simulink model "ramadan_2022"  (R2021a)
settings: Solver=ode15s  StartTime=0.0  StopTime=10  MaxStep=1e-2  MinStep=1e-20  RelTol=1e-3
StartFcn:
  | tic
StopFcn:
  | toc
  | 
  | 
  | %if GimbalLockFlag
  |  % fprintf(2, 'Almost reached Gimbal Lock of IMU. Simulation stopped.\n')
  | %end
  | 
  | %fprintf('Elapsed time: %4.2f sec (%4.2f%% realtime)\n', a, tout(end)/a*100)
values from neighbouring files (symbols this model uses):
  Balance = pMod(26:29)    [AssignSimulinkParams.m]    (also in assign_parameters.m = param(26:29))
  BalanceTrunkLat = pMod(22:25)    [AssignSimulinkParams.m]    (also in assign_parameters.m = param(22:25))
  BasisStim = pMod(1:11)    [AssignSimulinkParams.m]    (also in assign_parameters.m = param(1:11))
  CompliantLeg = pMod(12:14)    [AssignSimulinkParams.m]    (also in assign_parameters.m = param(12:14))
  CompliantLegLat = pMod(15)    [AssignSimulinkParams.m]    (also in assign_parameters.m = param(15))
  lp1 = 0.45    [nms3D_prep.m]
  lp2 = 0.55    [nms3D_prep.m]
  N = size(x,1)    [cmaes_hg.m]
  PreventKneeOverextension = pMod(16:21)    [AssignSimulinkParams.m]    (also in assign_parameters.m = param(16:21))
  propulsion = pMod(35)    [AssignSimulinkParams.m]    (also in assign_parameters.m = param(35))
  s = x(1:N-1,:).^2 + x(2:N,:).^2    [cmaes_hg.m]
  Target02 = pMod(30)    [AssignSimulinkParams.m]    (also in assign_parameters.m = param(30))
  Target13 = pMod(31:33)    [AssignSimulinkParams.m]    (also in assign_parameters.m = param(31:33))
  theta0 = pMod(34)    [AssignSimulinkParams.m]    (also in assign_parameters.m = param(34))
  WramameiSL_1000 = readmatrix('WSL_1000_Norm_Sigmoid_MSE_cont.csv')    [nms3D_prep.m]
  ZramameiSL_1000 = readmatrix('ZSL_1000_Norm_Sigmoid_MSE_cont.csv')    [nms3D_prep.m]
undefined symbols (not defined in the file or in its folder): ICs, mParams, X, Y, Z
libraries: nesl_utility x110, sm_lib x88, simulink x79, eeGeneralControl x28, robotmaniplib x10, dspinverses x10, robotcorelib x5, dspmathops x3, pid_lib x2, vrlib x1
(part 8 of 9)

== system ramadan_2022/Supraspinal Level/Subsystem/Swing Leg/Compute Acceleration Profiles with Minimal Jerk Approach/Minimal jerk Hip Roll ==
  T_tot : Inport
  t_passed : Inport  Port=2
  "x0, dx0, ddx0" : Inport  Port=3
  "xT, dxT, ddxT" : Inport  Port=4
  Compare To Constant : simulink/Logic and Bit Operations/Compare To Constant  relop=>=  const=mParams.control.timelimit  OutDataTypeStr=boolean  ZeroCross=off
  Constant : Constant  Value=mParams.control.timelimit
  Constant1 : Constant  Value=0
  Demux : Demux  Outputs=3
  Demux1 : Demux  Outputs=3
  Enabled Subsystem : Subsystem  TreatAsAtomicUnit=on
  Minimal Jerk : Subsystem
  Minimal Jerk Parameters [Movellan] : Subsystem
  Minus : Sum  Inputs=+-
  Minus1 : Sum  Inputs=+-
  Switch : Switch
  jerk : Outport
  wires:
  Minimal Jerk/1(j(t)) -> jerk/1
  T_tot/1 -> Minus/1
  t_passed/1 -> Minus/2
  Constant1/1 -> Switch/1
  Demux/1 -> Minimal Jerk Parameters [Movellan]/1(x0)
  Demux/2 -> Minimal Jerk Parameters [Movellan]/2(dx0)
  Demux/3 -> Minimal Jerk Parameters [Movellan]/3(ddx0)
  Demux1/1 -> Minimal Jerk Parameters [Movellan]/4(xT)
  "x0, dx0, ddx0"/1 -> Demux/1
  Demux1/2 -> Minimal Jerk Parameters [Movellan]/5(dxT)
  "xT, dxT, ddxT"/1 -> Demux1/1
  Demux1/3 -> Minimal Jerk Parameters [Movellan]/6(ddxT)
  Minimal Jerk Parameters [Movellan]/1(a) -> Enabled Subsystem/1(In1)
  Minus/1 -> Compare To Constant/1, Minus1/2, Minimal Jerk Parameters [Movellan]/7(T)
  Enabled Subsystem/1(Out1) -> Minimal Jerk/2(a [6x1])
  Compare To Constant/1 -> Switch/2, Enabled Subsystem/Enable
  Constant/1 -> Minus1/1
  Minus1/1 -> Switch/3
  Switch/1 -> Minimal Jerk/1(t)

== system ramadan_2022/Supraspinal Level/Subsystem/Swing Leg/Compute Acceleration Profiles with Minimal Jerk Approach/Minimal jerk Hip Roll4 ==
  T_tot : Inport
  t_passed : Inport  Port=2
  "x0, dx0, ddx0" : Inport  Port=3
  "xT, dxT, ddxT" : Inport  Port=4
  Constant1 : Constant  Value=0
  Demux : Demux  Outputs=3
  Demux1 : Demux  Outputs=3
  Minimal Jerk : Subsystem
  Minimal Jerk Parameters[Movellan] : Subsystem
  Minus : Sum  Inputs=+-
  Saturation : Saturate  UpperLimit=inf  LowerLimit=0.08
  jerk : Outport
  wires:
  Minimal Jerk/1(j(t)) -> jerk/1
  T_tot/1 -> Minus/1
  Minimal Jerk Parameters[Movellan]/1(a) -> Minimal Jerk/2(a [6x1])
  t_passed/1 -> Minus/2
  Constant1/1 -> Minimal Jerk/1(t)
  Minus/1 -> Saturation/1
  Demux/1 -> Minimal Jerk Parameters[Movellan]/1(x0)
  Demux/2 -> Minimal Jerk Parameters[Movellan]/2(dx0)
  Demux/3 -> Minimal Jerk Parameters[Movellan]/3(ddx0)
  Demux1/1 -> Minimal Jerk Parameters[Movellan]/4(xT)
  "x0, dx0, ddx0"/1 -> Demux/1
  Demux1/2 -> Minimal Jerk Parameters[Movellan]/5(dxT)
  "xT, dxT, ddxT"/1 -> Demux1/1
  Demux1/3 -> Minimal Jerk Parameters[Movellan]/6(ddxT)
  Saturation/1 -> Minimal Jerk Parameters[Movellan]/7(T)

== system ramadan_2022/Supraspinal Level/Subsystem/Swing Leg/Compute Acceleration Profiles with Minimal Jerk Approach/Minimal jerk Knee ==
  T_tot : Inport
  t_passed : Inport  Port=2
  "x0, dx0, ddx0" : Inport  Port=3
  "xT, dxT, ddxT" : Inport  Port=4
  Compare To Constant1 : simulink/Logic and Bit Operations/Compare To Constant  relop=>=  const=mParams.control.timelimit  OutDataTypeStr=boolean  ZeroCross=off
  Constant : Constant  Value=mParams.control.timelimit
  Constant1 : Constant  Value=0
  Demux : Demux  Outputs=3
  Demux1 : Demux  Outputs=3
  Enabled Subsystem : Subsystem  TreatAsAtomicUnit=on
  Minimal Jerk : Subsystem
  Minimal Jerk Parameters [Movellan] : Subsystem
  Minus : Sum  Inputs=+-
  Minus1 : Sum  Inputs=+-
  Scope : Scope
  Scope1 : Scope  NumInputPorts=2
  Scope2 : Scope
  Switch : Switch
  jerk : Outport
  wires:
  Minimal Jerk/1(j(t)) -> jerk/1
  T_tot/1 -> Minus/1
  t_passed/1 -> Minus/2
  Constant1/1 -> Switch/1
  Demux/1 -> Scope1/1, Minimal Jerk Parameters [Movellan]/1(x0)
  Demux/2 -> Minimal Jerk Parameters [Movellan]/2(dx0)
  Demux/3 -> Minimal Jerk Parameters [Movellan]/3(ddx0)
  Demux1/1 -> Scope1/2, Minimal Jerk Parameters [Movellan]/4(xT)
  "x0, dx0, ddx0"/1 -> Demux/1
  Demux1/2 -> Minimal Jerk Parameters [Movellan]/5(dxT)
  "xT, dxT, ddxT"/1 -> Demux1/1
  Demux1/3 -> Minimal Jerk Parameters [Movellan]/6(ddxT)
  Minimal Jerk Parameters [Movellan]/1(a) -> Enabled Subsystem/1(In1)
  Minus/1 -> Scope/1, Compare To Constant1/1, Minus1/2, Minimal Jerk Parameters [Movellan]/7(T)
  Enabled Subsystem/1(Out1) -> Minimal Jerk/2(a [6x1])
  Compare To Constant1/1 -> Switch/2, Enabled Subsystem/Enable
  Constant/1 -> Minus1/1
  Minus1/1 -> Switch/3
  Switch/1 -> Minimal Jerk/1(t)

== system ramadan_2022/Supraspinal Level/Subsystem/Swing Leg/Compute Acceleration Profiles with Minimal Jerk Approach1/ Timer Phase 1 ==
  R : Inport
  Clock1 : Clock
  Clock3 : Clock
      settings: Decimation=4
  NOT : Logic  Operator=NOT  AllPortsSameDT=off  OutDataTypeStr=boolean
  Resettable Subsystem : Subsystem  TreatAsAtomicUnit=on
  Sum1 : Sum  Inputs=|+-  InputSameDT=on  SaturateOnIntegerOverflow=on  OutDataTypeStr=Inherit: Same as first input
  Switch2 : Switch  Criteria=u2 > Threshold  RndMeth=Zero
  t_passed : Outport  VectorParamsAs1DForOutWhenUnconnected=off
  wires:
  Clock1/1 -> Sum1/1
  Clock3/1 -> Switch2/3, Resettable Subsystem/1(In1)
  Sum1/1 -> t_passed/1
  R/1 -> NOT/1, Switch2/2
  Switch2/1 -> Sum1/2
  Resettable Subsystem/1(Out1) -> Switch2/1
  NOT/1 -> Resettable Subsystem/Enable

== system ramadan_2022/Supraspinal Level/Subsystem/Swing Leg/Compute Acceleration Profiles with Minimal Jerk Approach1/ Timer Phase 2 ==
  R : Inport
  Clock1 : Clock
  Clock3 : Clock
      settings: Decimation=4
  NOT : Logic  Operator=NOT  AllPortsSameDT=off  OutDataTypeStr=boolean
  Resettable Subsystem : Subsystem  TreatAsAtomicUnit=on
  Sum1 : Sum  Inputs=|+-  InputSameDT=on  SaturateOnIntegerOverflow=on  OutDataTypeStr=Inherit: Same as first input
  Switch2 : Switch  Criteria=u2 > Threshold  RndMeth=Zero
  Out : Outport  VectorParamsAs1DForOutWhenUnconnected=off
  wires:
  Clock1/1 -> Sum1/1
  Clock3/1 -> Switch2/3, Resettable Subsystem/1(In1)
  Sum1/1 -> Out/1
  R/1 -> NOT/1, Switch2/2
  Switch2/1 -> Sum1/2
  Resettable Subsystem/1(Out1) -> Switch2/1
  NOT/1 -> Resettable Subsystem/Enable

== system ramadan_2022/Supraspinal Level/Subsystem/Swing Leg/Compute Acceleration Profiles with Minimal Jerk Approach1/ Timer Phase 3 ==
  R : Inport
  Clock1 : Clock
  Clock3 : Clock
      settings: Decimation=4
  NOT : Logic  Operator=NOT  AllPortsSameDT=off  OutDataTypeStr=boolean
  Resettable Subsystem : Subsystem  TreatAsAtomicUnit=on
  Sum1 : Sum  Inputs=|+-  InputSameDT=on  SaturateOnIntegerOverflow=on  OutDataTypeStr=Inherit: Same as first input
  Switch2 : Switch  Criteria=u2 > Threshold  RndMeth=Zero
  t_passed : Outport  VectorParamsAs1DForOutWhenUnconnected=off
  wires:
  Clock1/1 -> Sum1/1
  Clock3/1 -> Switch2/3, Resettable Subsystem/1(In1)
  Sum1/1 -> t_passed/1
  R/1 -> NOT/1, Switch2/2
  Switch2/1 -> Sum1/2
  Resettable Subsystem/1(Out1) -> Switch2/1
  NOT/1 -> Resettable Subsystem/Enable

== system ramadan_2022/Supraspinal Level/Subsystem/Swing Leg/Compute Acceleration Profiles with Minimal Jerk Approach1/ Timer Phase 4 ==
  R : Inport
  Clock1 : Clock
  Clock3 : Clock
      settings: Decimation=4
  NOT : Logic  Operator=NOT  AllPortsSameDT=off  OutDataTypeStr=boolean
  Resettable Subsystem : Subsystem  TreatAsAtomicUnit=on
  Sum1 : Sum  Inputs=|+-  InputSameDT=on  SaturateOnIntegerOverflow=on  OutDataTypeStr=Inherit: Same as first input
  Switch2 : Switch  Criteria=u2 > Threshold  RndMeth=Zero
  t_passed : Outport  VectorParamsAs1DForOutWhenUnconnected=off
  wires:
  Clock1/1 -> Sum1/1
  Clock3/1 -> Switch2/3, Resettable Subsystem/1(In1)
  Sum1/1 -> t_passed/1
  R/1 -> NOT/1, Switch2/2
  Switch2/1 -> Sum1/2
  Resettable Subsystem/1(Out1) -> Switch2/1
  NOT/1 -> Resettable Subsystem/Enable

== system ramadan_2022/Supraspinal Level/Subsystem/Swing Leg/Compute Acceleration Profiles with Minimal Jerk Approach1/Minimal jerk Hip Roll4 ==
  T_tot : Inport
  t_passed : Inport  Port=2
  "x0, dx0, ddx0" : Inport  Port=3
  "xT, dxT, ddxT" : Inport  Port=4
  Constant1 : Constant  Value=0
  Demux : Demux  Outputs=3
  Demux1 : Demux  Outputs=3
  Minimal Jerk : Subsystem
  Minimal Jerk Parameters[Movellan] : Subsystem
  Minus : Sum  Inputs=+-
  Saturation : Saturate  UpperLimit=inf  LowerLimit=0.08
  jerk : Outport
  wires:
  Minimal Jerk/1(j(t)) -> jerk/1
  T_tot/1 -> Minus/1
  Minimal Jerk Parameters[Movellan]/1(a) -> Minimal Jerk/2(a [6x1])
  t_passed/1 -> Minus/2
  Constant1/1 -> Minimal Jerk/1(t)
  Minus/1 -> Saturation/1
  Demux/1 -> Minimal Jerk Parameters[Movellan]/1(x0)
  Demux/2 -> Minimal Jerk Parameters[Movellan]/2(dx0)
  Demux/3 -> Minimal Jerk Parameters[Movellan]/3(ddx0)
  Demux1/1 -> Minimal Jerk Parameters[Movellan]/4(xT)
  "x0, dx0, ddx0"/1 -> Demux/1
  Demux1/2 -> Minimal Jerk Parameters[Movellan]/5(dxT)
  "xT, dxT, ddxT"/1 -> Demux1/1
  Demux1/3 -> Minimal Jerk Parameters[Movellan]/6(ddxT)
  Saturation/1 -> Minimal Jerk Parameters[Movellan]/7(T)

== system ramadan_2022/Supraspinal Level/Subsystem/Swing Leg/Compute Acceleration Profiles with Minimal Jerk Approach1/Minimal jerk Leg Angle ==
  T_tot : Inport
  t_passed : Inport  Port=2
  "x0, dx0, ddx0" : Inport  Port=3
  "xT, dxT, ddxT" : Inport  Port=4
  Compare To Constant : simulink/Logic and Bit Operations/Compare To Constant  relop=>=  const=mParams.control.timelimit  OutDataTypeStr=boolean  ZeroCross=off
  Constant : Constant  Value=mParams.control.timelimit
  Constant1 : Constant  Value=0
  Demux : Demux  Outputs=3
  Demux1 : Demux  Outputs=3
  Enabled Subsystem : Subsystem  TreatAsAtomicUnit=on
  Minimal Jerk : Subsystem
  Minimal Jerk Parameters [Movellan] : Subsystem
  Minus : Sum  Inputs=+-
  Minus1 : Sum  Inputs=+-
  Switch : Switch
  jerk : Outport
  wires:
  Minimal Jerk/1(j(t)) -> jerk/1
  T_tot/1 -> Minus/1
  t_passed/1 -> Minus/2
  Constant1/1 -> Switch/1
  Demux/1 -> Minimal Jerk Parameters [Movellan]/1(x0)
  Demux/2 -> Minimal Jerk Parameters [Movellan]/2(dx0)
  Demux/3 -> Minimal Jerk Parameters [Movellan]/3(ddx0)
  Demux1/1 -> Minimal Jerk Parameters [Movellan]/4(xT)
  "x0, dx0, ddx0"/1 -> Demux/1
  Demux1/2 -> Minimal Jerk Parameters [Movellan]/5(dxT)
  "xT, dxT, ddxT"/1 -> Demux1/1
  Demux1/3 -> Minimal Jerk Parameters [Movellan]/6(ddxT)
  Minimal Jerk Parameters [Movellan]/1(a) -> Enabled Subsystem/1(In1)
  Minus/1 -> Compare To Constant/1, Minus1/2, Minimal Jerk Parameters [Movellan]/7(T)
  Enabled Subsystem/1(Out1) -> Minimal Jerk/2(a [6x1])
  Compare To Constant/1 -> Switch/2, Enabled Subsystem/Enable
  Constant/1 -> Minus1/1
  Minus1/1 -> Switch/3
  Switch/1 -> Minimal Jerk/1(t)

== system ramadan_2022/Supraspinal Level/Subsystem/Swing Leg/Compute Acceleration Profiles with Minimal Jerk Approach1/Minimal jerk Leg Length ==
  T_tot : Inport
  t_passed : Inport  Port=2
  "x0, dx0, ddx0" : Inport  Port=3
  "xT, dxT, ddxT" : Inport  Port=4
  Compare To Constant1 : simulink/Logic and Bit Operations/Compare To Constant  relop=>=  const=mParams.control.timelimit  OutDataTypeStr=boolean  ZeroCross=off
  Constant : Constant  Value=mParams.control.timelimit
  Constant1 : Constant  Value=0
  Demux : Demux  Outputs=3
  Demux1 : Demux  Outputs=3
  Enabled Subsystem : Subsystem  TreatAsAtomicUnit=on
  Minimal Jerk : Subsystem
  Minimal Jerk Parameters [Movellan] : Subsystem
  Minus : Sum  Inputs=+-
  Minus1 : Sum  Inputs=+-
  Switch : Switch
  jerk : Outport
  wires:
  Minimal Jerk/1(j(t)) -> jerk/1
  T_tot/1 -> Minus/1
  t_passed/1 -> Minus/2
  Constant1/1 -> Switch/1
  Demux/1 -> Minimal Jerk Parameters [Movellan]/1(x0)
  Demux/2 -> Minimal Jerk Parameters [Movellan]/2(dx0)
  Demux/3 -> Minimal Jerk Parameters [Movellan]/3(ddx0)
  Demux1/1 -> Minimal Jerk Parameters [Movellan]/4(xT)
  "x0, dx0, ddx0"/1 -> Demux/1
  Demux1/2 -> Minimal Jerk Parameters [Movellan]/5(dxT)
  "xT, dxT, ddxT"/1 -> Demux1/1
  Demux1/3 -> Minimal Jerk Parameters [Movellan]/6(ddxT)
  Minimal Jerk Parameters [Movellan]/1(a) -> Enabled Subsystem/1(In1)
  Minus/1 -> Compare To Constant1/1, Minus1/2, Minimal Jerk Parameters [Movellan]/7(T)
  Enabled Subsystem/1(Out1) -> Minimal Jerk/2(a [6x1])
  Compare To Constant1/1 -> Switch/2, Enabled Subsystem/Enable
  Constant/1 -> Minus1/1
  Minus1/1 -> Switch/3
  Switch/1 -> Minimal Jerk/1(t)

== system ramadan_2022/Supraspinal Level/Subsystem/Swing Leg/Compute Target States/Balance Control lateral ==
  Left/Right : Inport
  Constant : Constant  Value=0
  Constant1 : Constant
  Constant2 : Constant  Value=-1
  Divide : Product  Inputs=**
  Divide1 : Product  Inputs=**
  Minus5 : Sum  Inputs=+++
  Minus6 : Sum  Inputs=+-
  Product : Product
  Selector3 : Selector  InputPortWidth=3  IndexOptions=Index vector (dialog)  Indices=[3]  OutputSizes=1
  Selector4 : Selector  InputPortWidth=3  IndexOptions=Index vector (dialog)  Indices=[3]  OutputSizes=1
  Selector5 : Selector  InputPortWidth=3  IndexOptions=Index vector (dialog)  Indices=[3]  OutputSizes=1
  Switch : Switch  Criteria=u2 > Threshold
  Switch1 : Switch  Criteria=u2 > Threshold
  theta_Hip_swing_target : Outport
  wires:
  Divide/1 -> Minus5/2
  Switch/1 -> Minus6/2
  Divide1/1 -> Minus5/3
  [AnklePosR_rot] -> Selector3/1
  Minus6/1 -> Divide1/1
  Left/Right/1 -> Switch1/2, Switch/2
  [AnklePosL_rot] -> Selector4/1
  [cv_lat] -> Divide/2
  [cd_lat] -> Divide1/2
  Selector4/1 -> Switch/1
  Selector3/1 -> Switch/3
  [CoM_Velocity_rot] -> Selector5/1
  Selector5/1 -> Divide/1
  Constant/1 -> Minus6/1
  Minus5/1 -> theta_Hip_swing_target/1
  Product/1 -> Minus5/1
  [swh_lat] -> Product/2
  Switch1/1 -> Product/1
  Constant1/1 -> Switch1/1
  Constant2/1 -> Switch1/3

== system ramadan_2022/Supraspinal Level/Subsystem/Swing Leg/Compute Target States/Balance Control saggital ==
  Left/Right : Inport
  Constant : Constant  Value=0
  Divide : Product  Inputs=**
  Divide1 : Product  Inputs=**
  Minus5 : Sum  Inputs=+++
  Minus6 : Sum  Inputs=+-
  Selector3 : Selector  InputPortWidth=3  IndexOptions=Index vector (dialog)  Indices=[1]  OutputSizes=1
  Selector4 : Selector  InputPortWidth=3  IndexOptions=Index vector (dialog)  Indices=[1]  OutputSizes=1
  Selector5 : Selector  InputPortWidth=3  IndexOptions=Index vector (dialog)  Indices=[1]  OutputSizes=1
  Switch : Switch  Criteria=u2 > Threshold
  theta_Hip_swing_target : Outport
  tag scope: d=global
  wires:
  [swh] -> Minus5/1
  Switch/1 -> Minus6/2
  [AnklePosR_rot] -> Selector4/1
  Minus6/1 -> [d], Divide1/1
  Left/Right/1 -> Switch/2
  [AnklePosL_rot] -> Selector3/1
  [cv] -> Divide/2
  [cd] -> Divide1/2
  Divide/1 -> Minus5/2
  [CoM_Velocity_rot] -> Selector5/1
  Constant/1 -> Minus6/1
  Divide1/1 -> Minus5/3
  Minus5/1 -> theta_Hip_swing_target/1
  Selector5/1 -> Divide/1
  Selector3/1 -> Switch/1
  Selector4/1 -> Switch/3

== system ramadan_2022/Supraspinal Level/Subsystem/Swing Leg/Inverse Dynamics: Left Leg/Inverse Dynamics ==
  note: Augment Joint Vectors: In order to compute appropriate gravitational and velocity dependend forces, the joint angle and joint angle acceleration vectors are augmented by the position and velocity of the body in space.
  Joint Angles [rad] : Inport
  Joint Angle Velocities [rad/s] : Inport  Port=2
  Joint  Acceleration [rad/s^2] : Inport  Port=3
  Rotation Trunk [rad] : Inport  Port=4
  Trunk Position [m] : Inport  Port=5
  Rotation Velocity Trunk [rad/s] : Inport  Port=6
  Trunk Velocity [m/s] : Inport  Port=7
  Desired Acceleration [rad/s^2] : Inport  Port=8
  Enable : EnablePort  ZeroCross=off
  Constant : Constant  Value=zeros(6,1)
  Inverse Dynamics : Subsystem
  Mux : Mux  Inputs=3
  Mux1 : Mux  Inputs=3
  Mux2 : Mux  Inputs=2
  Mux4 : Mux  Inputs=2
  " Desired Torques" : Outport  VectorParamsAs1DForOutWhenUnconnected=off
  Interaction Wrench : Outport  Port=2  VectorParamsAs1DForOutWhenUnconnected=off
  wires:
  Trunk Position [m]/1 -> Mux1/1
  Inverse Dynamics/1(Desired Torques) -> " Desired Torques"/1
  Mux1/1 -> Inverse Dynamics/1(Config)
  Joint Angles [rad]/1 -> Mux1/3
  Rotation Trunk [rad]/1 -> Mux1/2
  Joint Angle Velocities [rad/s]/1 -> Mux/3
  Mux/1 -> Inverse Dynamics/2(JointVel)
  Desired Acceleration [rad/s^2]/1 -> Mux2/2
  Mux2/1 -> Inverse Dynamics/3(Des. JointAccel)
  Inverse Dynamics/2(Interaction Wrench Left) -> Interaction Wrench/1
  Constant/1 -> Mux4/1, Mux2/1
  Mux4/1 -> Inverse Dynamics/4(Real JointAccel)
  Joint  Acceleration [rad/s^2]/1 -> Mux4/2
  Trunk Velocity [m/s]/1 -> Mux/1
  Rotation Velocity Trunk [rad/s]/1 -> Mux/2

== system ramadan_2022/Supraspinal Level/Subsystem/Swing Leg/Inverse Dynamics: Left Leg/Sensor Data from Body Layer ==
  Constant : Constant  Commented=on  Value=0
  Constant1 : Constant  Value=zeros(3,1)
  From3 : From  Commented=on  GotoTag=TrunkRot_lat  TagVisibility=global
  From4 : From  Commented=on  GotoTag=TrunkRot_sag  TagVisibility=global
  From44 : From  Commented=on  GotoTag=RotationalVelocityTrunk  TagVisibility=global
  From46 : From  Commented=on  GotoTag=TranslationalVelocityTrunk  TagVisibility=global
  Gain : Gain  Gain=0
  Gain1 : Gain  Gain=0
  Mux : Mux  Commented=on  Inputs=3
  Scope : Scope
  Sensor Delay 1 : eeGeneralControl/Low-Pass Filter (Discrete or Continuous)  K=1  T=0.01  B=inf  A=-inf  init_option=Inherited from block input  x0=0  Ts=-1
  Sensor Delay 2 : eeGeneralControl/Low-Pass Filter (Discrete or Continuous)  K=1  T=0.01  B=inf  A=-inf  init_option=Inherited from block input  x0=0  Ts=-1
  Sensor Delay 3 : eeGeneralControl/Low-Pass Filter (Discrete or Continuous)  K=1  T=0.01  B=inf  A=-inf  init_option=Inherited from block input  x0=0  Ts=-1
  Joint Angles [rad] : Outport
  Joint Angle Velocities [rad/s] : Outport  Port=2
  Joint Angle Accelerations [rad/s^2] : Outport  Port=3
  " Rotation Trunk [rad]" : Outport  Port=4
  Trunk Position [m] : Outport  Port=5
  Rotation Velocity Trunk [rad/s] : Outport  Port=6
  Trunk Velocity [m/s] : Outport  Port=7
  wires:
  [Llegq] -> Sensor Delay 3/1
  [Llegdq] -> Sensor Delay 1/1
  Sensor Delay 3/1 -> Joint Angles [rad]/1
  Sensor Delay 1/1 -> Joint Angle Velocities [rad/s]/1
  [CoM_Position] -> Trunk Position [m]/1
  [Llegddq] -> Sensor Delay 2/1
  Sensor Delay 2/1 -> Joint Angle Accelerations [rad/s^2]/1, Scope/1
  From3/1 -> Mux/1
  Constant/1 -> Mux/2
  From4/1 -> Mux/3
  [RotationTrunk] -> " Rotation Trunk [rad]"/1
  Gain/1 -> Rotation Velocity Trunk [rad/s]/1
  Gain1/1 -> Trunk Velocity [m/s]/1
  Constant1/1 -> Gain1/1, Gain/1

== system ramadan_2022/Supraspinal Level/Subsystem/Swing Leg/Inverse Dynamics: Right Leg/Inverse Dynamics1 ==
  note: Augment Joint Vectors: In order to compute appropriate gravitational and velocity dependend forces, the joint angle and joint angle acceleration vectors are augmented by the position and velocity of the body in space.
  Joint Angles [rad] : Inport
  Joint Angle Velocities [rad/s] : Inport  Port=2
  Joint  Acceleration [rad/s^2] : Inport  Port=3
  Rotation Trunk [rad] : Inport  Port=4
  Trunk Position [m] : Inport  Port=5
  Rotation Velocity Trunk [rad/s] : Inport  Port=6
  Trunk Velocity [m/s] : Inport  Port=7
  Desired Acceleration [rad/s^2] : Inport  Port=8
  Enable : EnablePort  ZeroCross=off
  Constant : Constant  Value=zeros(6,1)
  Inverse Dynamics : Subsystem
  Mux : Mux  Inputs=3
  Mux1 : Mux  Inputs=3
  Mux2 : Mux  Inputs=2
  Mux4 : Mux  Inputs=2
  " Desired Torques" : Outport  VectorParamsAs1DForOutWhenUnconnected=off
  Interaction Wrench : Outport  Port=2  VectorParamsAs1DForOutWhenUnconnected=off
  wires:
  Trunk Position [m]/1 -> Mux1/1
  Inverse Dynamics/1(Desired Torques) -> " Desired Torques"/1
  Mux1/1 -> Inverse Dynamics/1(Config)
  Joint Angles [rad]/1 -> Mux1/3
  Rotation Trunk [rad]/1 -> Mux1/2
  Joint Angle Velocities [rad/s]/1 -> Mux/3
  Mux/1 -> Inverse Dynamics/2(JointVel)
  Desired Acceleration [rad/s^2]/1 -> Mux2/2
  Mux2/1 -> Inverse Dynamics/3(Des. JointAccel)
  Constant/1 -> Mux4/1, Mux2/1
  Mux4/1 -> Inverse Dynamics/4(Real JointAccel)
  Joint  Acceleration [rad/s^2]/1 -> Mux4/2
  Inverse Dynamics/2(Interaction Wrench Left) -> Interaction Wrench/1
  Trunk Velocity [m/s]/1 -> Mux/1
  Rotation Velocity Trunk [rad/s]/1 -> Mux/2

== system ramadan_2022/Supraspinal Level/Subsystem/Swing Leg/Inverse Dynamics: Right Leg/Sensor Data from Body Layer1 ==
  Constant1 : Constant  Value=zeros(3,1)
  From44 : From  Commented=on  GotoTag=RotationalVelocityTrunk  TagVisibility=global
  From46 : From  Commented=on  GotoTag=TranslationalVelocityTrunk  TagVisibility=global
  Gain : Gain  Gain=0
  Gain1 : Gain  Gain=0
  Sensor Delay 1 : eeGeneralControl/Low-Pass Filter (Discrete or Continuous)  K=1  T=0.01  B=inf  A=-inf  init_option=Inherited from block input  x0=0  Ts=-1
  Sensor Delay 2 : eeGeneralControl/Low-Pass Filter (Discrete or Continuous)  K=1  T=0.01  B=inf  A=-inf  init_option=Inherited from block input  x0=0  Ts=-1
  Sensor Delay 3 : eeGeneralControl/Low-Pass Filter (Discrete or Continuous)  K=1  T=0.01  B=inf  A=-inf  init_option=Inherited from block input  x0=0  Ts=-1
  Joint Angles [rad] : Outport
  Joint Angle Velocities [rad/s] : Outport  Port=2
  Joint Angle Accelerations [rad/s^2] : Outport  Port=3
  " Rotation Trunk [rad]" : Outport  Port=4
  Trunk Position [m] : Outport  Port=5
  Rotation Velocity Trunk [rad/s] : Outport  Port=6
  Trunk Velocity [m/s] : Outport  Port=7
  wires:
  [Rlegq] -> Sensor Delay 3/1
  [Rlegdq] -> Sensor Delay 1/1
  Sensor Delay 3/1 -> Joint Angles [rad]/1
  Sensor Delay 1/1 -> Joint Angle Velocities [rad/s]/1
  [CoM_Position] -> Trunk Position [m]/1
  [Rlegddq] -> Sensor Delay 2/1
  Sensor Delay 2/1 -> Joint Angle Accelerations [rad/s^2]/1
  [RotationTrunk] -> " Rotation Trunk [rad]"/1
  Gain/1 -> Rotation Velocity Trunk [rad/s]/1
  Gain1/1 -> Trunk Velocity [m/s]/1
  Constant1/1 -> Gain1/1, Gain/1

== system ramadan_2022/Supraspinal Level/Subsystem/Stance Leg2/Stance Leg/Inverse Dynamics Left Leg/Left Leg Ball ==
  Config : Inport
  Task : Inport  Port=2
  PD Input : Inport  Port=3
  Enable : EnablePort  ZeroCross=off
  Constant1 : Constant  Value="[0 0   ]"
  Gain : Gain
  Get Jacobian : robotmaniplib/Get Jacobian  RigidBodyTree=model_left_ball  EndEffector=EEF  SimulateUsing=Code generation
      settings: SourceProductBaseCode=RO
  Joint Space Mass Matrix : robotmaniplib/Joint Space Mass Matrix  RigidBodyTree=model_left_ball  SimulateUsing=Code generation
  Matrix Concatenate : Concatenate  Mode=Multidimensional array
  Matrix Multiply1 : Product  Multiplication=Matrix(*)
  Matrix Multiply4 : Product  Multiplication=Matrix(*)
  Mux2 : Mux  Inputs=3
  Pseudoinverse1 : dspinverses/Pseudoinverse  wanterr=off  SimulateUsing=Code generation
      settings: SourceProductBaseCode=DS
  Selector2 : Selector  NumberOfDimensions=2  InputPortWidth=3  IndexOptions=Index vector (dialog),Index vector (dialog)  Indices=mParams.control.constraints.pushoff,[1:5]  OutputSizes=1,1
  Selector3 : Selector  NumberOfDimensions=2  InputPortWidth=3  IndexOptions=Index vector (dialog),Index vector (dialog)  Indices="[1  4 ],[1:5]"  OutputSizes=1,1
  Push-Off Left (Ball) : Outport
  wires:
  Config/1 -> Get Jacobian/1, Joint Space Mass Matrix/1
  Selector2/1 -> Matrix Concatenate/1
  Pseudoinverse1/1 -> Matrix Multiply4/1
  Matrix Concatenate/1 -> Pseudoinverse1/1
  Selector3/1 -> Matrix Concatenate/2
  Constant1/1 -> Mux2/3
  Mux2/1 -> Matrix Multiply4/2
  Matrix Multiply1/1 -> Push-Off Left (Ball)/1
  Joint Space Mass Matrix/1 -> Matrix Multiply1/1, Selector3/1
  Get Jacobian/1 -> Selector2/1
  PD Input/1 -> Gain/1
  Matrix Multiply4/1 -> Matrix Multiply1/2
  Task/1 -> Mux2/1
  Gain/1 -> Mux2/2

== system ramadan_2022/Supraspinal Level/Subsystem/Stance Leg2/Stance Leg/Subsystem/Right Leg Ball ==
  Config : Inport
  Task : Inport  Port=2
  PD : Inport  Port=3
  Enable : EnablePort  ZeroCross=off
  Constant1 : Constant  Value="[0 0  ]"
  Get Jacobian : robotmaniplib/Get Jacobian  RigidBodyTree=model_right_ball  EndEffector=EEF  SimulateUsing=Code generation
      settings: SourceProductBaseCode=RO
  Joint Space Mass Matrix : robotmaniplib/Joint Space Mass Matrix  RigidBodyTree=model_right_ball  SimulateUsing=Code generation
  Matrix Concatenate : Concatenate  Mode=Multidimensional array
  Matrix Multiply1 : Product  Multiplication=Matrix(*)
  Matrix Multiply4 : Product  Multiplication=Matrix(*)
  Mux2 : Mux  Inputs=3
  Pseudoinverse1 : dspinverses/Pseudoinverse  wanterr=off  SimulateUsing=Code generation
      settings: SourceProductBaseCode=DS
  Selector2 : Selector  NumberOfDimensions=2  InputPortWidth=3  IndexOptions=Index vector (dialog),Index vector (dialog)  Indices=mParams.control.constraints.pushoff,[1:5]  OutputSizes=1,1
  Selector3 : Selector  NumberOfDimensions=2  InputPortWidth=3  IndexOptions=Index vector (dialog),Index vector (dialog)  Indices="[1  4 ],[1:5]"  OutputSizes=1,1
  Push-Off Right (Ball) : Outport
  wires:
  Matrix Multiply4/1 -> Matrix Multiply1/2
  Config/1 -> Get Jacobian/1, Joint Space Mass Matrix/1
  Selector2/1 -> Matrix Concatenate/1
  Pseudoinverse1/1 -> Matrix Multiply4/1
  Matrix Concatenate/1 -> Pseudoinverse1/1
  Selector3/1 -> Matrix Concatenate/2
  Constant1/1 -> Mux2/3
  Mux2/1 -> Matrix Multiply4/2
  Matrix Multiply1/1 -> Push-Off Right (Ball)/1
  Get Jacobian/1 -> Selector2/1
  Joint Space Mass Matrix/1 -> Matrix Multiply1/1, Selector3/1
  PD/1 -> Mux2/2
  Task/1 -> Mux2/1

== system ramadan_2022/Supraspinal Level/Subsystem/Swing Leg/Compute Acceleration Profiles with Minimal Jerk Approach/ Timer Phase 1/Resettable Subsystem ==
  In1 : Inport
  Enable : EnablePort  ZeroCross=off
  Out1 : Outport
  wires:
  In1/1 -> Out1/1

== system ramadan_2022/Supraspinal Level/Subsystem/Swing Leg/Compute Acceleration Profiles with Minimal Jerk Approach/ Timer Phase 2/Resettable Subsystem ==
  In1 : Inport
  Enable : EnablePort  ZeroCross=off
  Out1 : Outport
  wires:
  In1/1 -> Out1/1

== system ramadan_2022/Supraspinal Level/Subsystem/Swing Leg/Compute Acceleration Profiles with Minimal Jerk Approach/ Timer Phase 3/Resettable Subsystem ==
  In1 : Inport
  Enable : EnablePort  ZeroCross=off
  Out1 : Outport
  wires:
  In1/1 -> Out1/1

== system ramadan_2022/Supraspinal Level/Subsystem/Swing Leg/Compute Acceleration Profiles with Minimal Jerk Approach/ Timer Phase 4/Resettable Subsystem ==
  In1 : Inport
  Enable : EnablePort  ZeroCross=off
  Out1 : Outport
  wires:
  In1/1 -> Out1/1

== system ramadan_2022/Supraspinal Level/Subsystem/Swing Leg/Compute Acceleration Profiles with Minimal Jerk Approach/Minimal jerk Ankle/Enabled Subsystem ==
  In1 : Inport
  Enable : EnablePort
  Out1 : Outport  VectorParamsAs1DForOutWhenUnconnected=off
  wires:
  In1/1 -> Out1/1

== system ramadan_2022/Supraspinal Level/Subsystem/Swing Leg/Compute Acceleration Profiles with Minimal Jerk Approach/Minimal jerk Ankle/Minimal Jerk ==
  t : Inport
  a [6x1] : Inport  Port=2
  Add : Sum  Inputs=3
  Constant1 : Constant
  Constant3 : Constant  Value=2
  Demux : Demux  Outputs=6
  Divide3 : Product  Inputs=**
  Divide4 : Product  Inputs=**
  Divide5 : Product  Inputs=**
  Gain : Gain  Gain=60
  Gain1 : Gain  Gain=24
  Gain2 : Gain  Gain=6
  Math Function4 : Math  Operator=pow  SaturateOnIntegerOverflow=on
  Terminator : Terminator
  Terminator1 : Terminator
  Terminator2 : Terminator
  j(t) : Outport
  wires:
  a [6x1]/1 -> Demux/1
  Constant3/1 -> Math Function4/2
  Add/1 -> j(t)/1
  Demux/4 -> Divide3/2
  t/1 -> Divide4/1, Math Function4/1
  Demux/5 -> Divide4/2
  Demux/6 -> Divide5/2
  Demux/1 -> Terminator/1
  Demux/2 -> Terminator1/1
  Divide3/1 -> Gain2/1
  Divide4/1 -> Gain1/1
  Divide5/1 -> Gain/1
  Gain/1 -> Add/3
  Gain1/1 -> Add/2
  Gain2/1 -> Add/1
  Math Function4/1 -> Divide5/1
  Constant1/1 -> Divide3/1
  Demux/3 -> Terminator2/1

== system ramadan_2022/Supraspinal Level/Subsystem/Swing Leg/Compute Acceleration Profiles with Minimal Jerk Approach/Minimal jerk Ankle/Minimal Jerk Parameters [Movellan] ==
  x0 : Inport
  dx0 : Inport  Port=2
  ddx0 : Inport  Port=3
  xT : Inport  Port=4
  dxT : Inport  Port=5
  ddxT : Inport  Port=6
  T : Inport  Port=7
  Demux : Demux  Outputs=3
  Gain : Gain  Gain=0.5
  Gain1 : Gain  Gain=3
  Gain2 : Gain  Gain=6
  Gain3 : Gain  Gain=4
  Gain4 : Gain  Gain=12
  Gain5 : Gain  Gain=5
  Gain6 : Gain  Gain=20
  Matrix Multiply : Product  Multiplication=Matrix(*)
  Minus : Sum  Inputs=+---
  Minus1 : Sum  Inputs=+--
  Minus2 : Sum  Inputs=+-
  Mux : Mux  Inputs=6
  Mux{1..4} (4 alike) : Mux  Inputs=3
  Pseudoinverse : dspinverses/Pseudoinverse  wanterr=off  SimulateUsing=Code generation
      settings: SourceProductBaseCode=DS
  T{2..5} (4 alike) : Product  Inputs=**
  b : Concatenate  NumInputs=3  Mode=Multidimensional array  ConcatenateDimension=2
  multiply : Product  Inputs=**
  multiply1 : Product  Inputs=**
  multiply2 : Product  Inputs=**
  a : Outport
  wires:
  xT/1 -> Minus/1
  Minus1/1 -> Mux4/2
  T5/1 -> Mux3/1
  multiply1/1 -> Minus1/3
  Gain5/1 -> Mux3/2
  Demux/2 -> Mux/5
  dxT/1 -> Minus1/1
  Demux/3 -> Mux/6
  b/1 -> Pseudoinverse/1
  multiply2/1 -> Minus/3
  Minus2/1 -> Mux4/3
  Gain/1 -> multiply/1, Mux/3
  multiply/1 -> Minus/4
  ddxT/1 -> Minus2/1
  Gain4/1 -> Mux2/3
  Gain6/1 -> Mux3/3
  x0/1 -> Minus/2, Mux/1
  Mux1/1 -> b/1
  Matrix Multiply/1 -> Demux/1
  ddx0/1 -> Minus2/2, multiply1/1, Gain/1
  T2/1 -> Gain1/1, Gain4/1, T3/1, multiply/2
  Gain2/1 -> Mux1/3
  Mux4/1 -> Matrix Multiply/2
  T4/1 -> Mux2/1, Gain5/1, T5/1
  Minus/1 -> Mux4/1
  Pseudoinverse/1 -> Matrix Multiply/1
  Mux2/1 -> b/2
  Gain3/1 -> Mux2/2
  Mux3/1 -> b/3
  Gain1/1 -> Mux1/2
  T/1 -> multiply2/2, multiply1/2, Gain2/1, T5/2, T4/2, T3/2, T2/2, T2/1
  Demux/1 -> Mux/4
  Mux/1 -> a/1
  T3/1 -> Gain6/1, Gain3/1, Mux1/1, T4/1
  dx0/1 -> multiply2/1, Minus1/2, Mux/2

== system ramadan_2022/Supraspinal Level/Subsystem/Swing Leg/Compute Acceleration Profiles with Minimal Jerk Approach/Minimal jerk Hip Pitch/Enabled Subsystem ==
  In1 : Inport
  Enable : EnablePort
  Out1 : Outport  VectorParamsAs1DForOutWhenUnconnected=off
  wires:
  In1/1 -> Out1/1

== system ramadan_2022/Supraspinal Level/Subsystem/Swing Leg/Compute Acceleration Profiles with Minimal Jerk Approach/Minimal jerk Hip Pitch/Minimal Jerk ==
  t : Inport
  a [6x1] : Inport  Port=2
  Add : Sum  Inputs=3
  Constant1 : Constant
  Constant3 : Constant  Value=2
  Demux : Demux  Outputs=6
  Divide3 : Product  Inputs=**
  Divide4 : Product  Inputs=**
  Divide5 : Product  Inputs=**
  Gain : Gain  Gain=60
  Gain1 : Gain  Gain=24
  Gain2 : Gain  Gain=6
  Math Function4 : Math  Operator=pow  SaturateOnIntegerOverflow=on
  Terminator : Terminator
  Terminator1 : Terminator
  Terminator2 : Terminator
  j(t) : Outport
  wires:
  a [6x1]/1 -> Demux/1
  Constant3/1 -> Math Function4/2
  Add/1 -> j(t)/1
  Demux/4 -> Divide3/2
  t/1 -> Divide4/1, Math Function4/1
  Demux/5 -> Divide4/2
  Demux/6 -> Divide5/2
  Demux/1 -> Terminator/1
  Demux/2 -> Terminator1/1
  Divide3/1 -> Gain2/1
  Divide4/1 -> Gain1/1
  Divide5/1 -> Gain/1
  Gain/1 -> Add/3
  Gain1/1 -> Add/2
  Gain2/1 -> Add/1
  Math Function4/1 -> Divide5/1
  Constant1/1 -> Divide3/1
  Demux/3 -> Terminator2/1

== system ramadan_2022/Supraspinal Level/Subsystem/Swing Leg/Compute Acceleration Profiles with Minimal Jerk Approach/Minimal jerk Hip Pitch/Minimal Jerk Parameters [Movellan] ==
  x0 : Inport
  dx0 : Inport  Port=2
  ddx0 : Inport  Port=3
  xT : Inport  Port=4
  dxT : Inport  Port=5
  ddxT : Inport  Port=6
  T : Inport  Port=7
  Demux : Demux  Outputs=3
  Gain : Gain  Gain=0.5
  Gain1 : Gain  Gain=3
  Gain2 : Gain  Gain=6
  Gain3 : Gain  Gain=4
  Gain4 : Gain  Gain=12
  Gain5 : Gain  Gain=5
  Gain6 : Gain  Gain=20
  Matrix Multiply : Product  Multiplication=Matrix(*)
  Minus : Sum  Inputs=+---
  Minus1 : Sum  Inputs=+--
  Minus2 : Sum  Inputs=+-
  Mux : Mux  Inputs=6
  Mux{1..4} (4 alike) : Mux  Inputs=3
  Pseudoinverse : dspinverses/Pseudoinverse  wanterr=off  SimulateUsing=Code generation
      settings: SourceProductBaseCode=DS
  T{2..5} (4 alike) : Product  Inputs=**
  b : Concatenate  NumInputs=3  Mode=Multidimensional array  ConcatenateDimension=2
  multiply : Product  Inputs=**
  multiply1 : Product  Inputs=**
  multiply2 : Product  Inputs=**
  a : Outport
  wires:
  xT/1 -> Minus/1
  Minus1/1 -> Mux4/2
  T5/1 -> Mux3/1
  multiply1/1 -> Minus1/3
  Gain5/1 -> Mux3/2
  Demux/2 -> Mux/5
  dxT/1 -> Minus1/1
  Demux/3 -> Mux/6
  b/1 -> Pseudoinverse/1
  multiply2/1 -> Minus/3
  Minus2/1 -> Mux4/3
  Gain/1 -> multiply/1, Mux/3
  multiply/1 -> Minus/4
  ddxT/1 -> Minus2/1
  Gain4/1 -> Mux2/3
  Gain6/1 -> Mux3/3
  x0/1 -> Minus/2, Mux/1
  Mux1/1 -> b/1
  Matrix Multiply/1 -> Demux/1
  ddx0/1 -> Minus2/2, multiply1/1, Gain/1
  T2/1 -> Gain1/1, Gain4/1, T3/1, multiply/2
  Gain2/1 -> Mux1/3
  Mux4/1 -> Matrix Multiply/2
  T4/1 -> Mux2/1, Gain5/1, T5/1
  Minus/1 -> Mux4/1
  Pseudoinverse/1 -> Matrix Multiply/1
  Mux2/1 -> b/2
  Gain3/1 -> Mux2/2
  Mux3/1 -> b/3
  Gain1/1 -> Mux1/2
  T/1 -> multiply2/2, multiply1/2, Gain2/1, T5/2, T4/2, T3/2, T2/2, T2/1
  Demux/1 -> Mux/4
  Mux/1 -> a/1
  T3/1 -> Gain6/1, Gain3/1, Mux1/1, T4/1
  dx0/1 -> multiply2/1, Minus1/2, Mux/2

== system ramadan_2022/Supraspinal Level/Subsystem/Swing Leg/Compute Acceleration Profiles with Minimal Jerk Approach/Minimal jerk Hip Roll/Enabled Subsystem ==
  In1 : Inport
  Enable : EnablePort
  Out1 : Outport  VectorParamsAs1DForOutWhenUnconnected=off
  wires:
  In1/1 -> Out1/1

== system ramadan_2022/Supraspinal Level/Subsystem/Swing Leg/Compute Acceleration Profiles with Minimal Jerk Approach/Minimal jerk Hip Roll/Minimal Jerk ==
  t : Inport
  a [6x1] : Inport  Port=2
  Add : Sum  Inputs=3
  Constant1 : Constant
  Constant3 : Constant  Value=2
  Demux : Demux  Outputs=6
  Divide3 : Product  Inputs=**
  Divide4 : Product  Inputs=**
  Divide5 : Product  Inputs=**
  Gain : Gain  Gain=60
  Gain1 : Gain  Gain=24
  Gain2 : Gain  Gain=6
  Math Function4 : Math  Operator=pow  SaturateOnIntegerOverflow=on
  Terminator : Terminator
  Terminator1 : Terminator
  Terminator2 : Terminator
  j(t) : Outport
  wires:
  a [6x1]/1 -> Demux/1
  Constant3/1 -> Math Function4/2
  Add/1 -> j(t)/1
  Demux/4 -> Divide3/2
  t/1 -> Divide4/1, Math Function4/1
  Demux/5 -> Divide4/2
  Demux/6 -> Divide5/2
  Demux/1 -> Terminator/1
  Demux/2 -> Terminator1/1
  Divide3/1 -> Gain2/1
  Divide4/1 -> Gain1/1
  Divide5/1 -> Gain/1
  Gain/1 -> Add/3
  Gain1/1 -> Add/2
  Gain2/1 -> Add/1
  Math Function4/1 -> Divide5/1
  Constant1/1 -> Divide3/1
  Demux/3 -> Terminator2/1

== system ramadan_2022/Supraspinal Level/Subsystem/Swing Leg/Compute Acceleration Profiles with Minimal Jerk Approach/Minimal jerk Hip Roll/Minimal Jerk Parameters [Movellan] ==
  x0 : Inport
  dx0 : Inport  Port=2
  ddx0 : Inport  Port=3
  xT : Inport  Port=4
  dxT : Inport  Port=5
  ddxT : Inport  Port=6
  T : Inport  Port=7
  Demux : Demux  Outputs=3
  Gain : Gain  Gain=0.5
  Gain1 : Gain  Gain=3
  Gain2 : Gain  Gain=6
  Gain3 : Gain  Gain=4
  Gain4 : Gain  Gain=12
  Gain5 : Gain  Gain=5
  Gain6 : Gain  Gain=20
  Matrix Multiply : Product  Multiplication=Matrix(*)
  Minus : Sum  Inputs=+---
  Minus1 : Sum  Inputs=+--
  Minus2 : Sum  Inputs=+-
  Mux : Mux  Inputs=6
  Mux{1..4} (4 alike) : Mux  Inputs=3
  Pseudoinverse : dspinverses/Pseudoinverse  wanterr=off  SimulateUsing=Code generation
      settings: SourceProductBaseCode=DS
  T{2..5} (4 alike) : Product  Inputs=**
  b : Concatenate  NumInputs=3  Mode=Multidimensional array  ConcatenateDimension=2
  multiply : Product  Inputs=**
  multiply1 : Product  Inputs=**
  multiply2 : Product  Inputs=**
  a : Outport
  wires:
  xT/1 -> Minus/1
  Minus1/1 -> Mux4/2
  T5/1 -> Mux3/1
  multiply1/1 -> Minus1/3
  Gain5/1 -> Mux3/2
  Demux/2 -> Mux/5
  dxT/1 -> Minus1/1
  Demux/3 -> Mux/6
  b/1 -> Pseudoinverse/1
  multiply2/1 -> Minus/3
  Minus2/1 -> Mux4/3
  Gain/1 -> multiply/1, Mux/3
  multiply/1 -> Minus/4
  ddxT/1 -> Minus2/1
  Gain4/1 -> Mux2/3
  Gain6/1 -> Mux3/3
  x0/1 -> Minus/2, Mux/1
  Mux1/1 -> b/1
  Matrix Multiply/1 -> Demux/1
  ddx0/1 -> Minus2/2, multiply1/1, Gain/1
  T2/1 -> Gain1/1, Gain4/1, T3/1, multiply/2
  Gain2/1 -> Mux1/3
  Mux4/1 -> Matrix Multiply/2
  T4/1 -> Mux2/1, Gain5/1, T5/1
  Minus/1 -> Mux4/1
  Pseudoinverse/1 -> Matrix Multiply/1
  Mux2/1 -> b/2
  Gain3/1 -> Mux2/2
  Mux3/1 -> b/3
  Gain1/1 -> Mux1/2
  T/1 -> multiply2/2, multiply1/2, Gain2/1, T5/2, T4/2, T3/2, T2/2, T2/1
  Demux/1 -> Mux/4
  Mux/1 -> a/1
  T3/1 -> Gain6/1, Gain3/1, Mux1/1, T4/1
  dx0/1 -> multiply2/1, Minus1/2, Mux/2

== system ramadan_2022/Supraspinal Level/Subsystem/Swing Leg/Compute Acceleration Profiles with Minimal Jerk Approach/Minimal jerk Hip Roll4/Minimal Jerk ==
  t : Inport
  a [6x1] : Inport  Port=2
  Add : Sum  Inputs=3
  Constant1 : Constant
  Constant3 : Constant  Value=2
  Demux : Demux  Outputs=6
  Divide3 : Product  Inputs=**
  Divide4 : Product  Inputs=**
  Divide5 : Product  Inputs=**
  Gain : Gain  Gain=60
  Gain1 : Gain  Gain=24
  Gain2 : Gain  Gain=6
  Math Function4 : Math  Operator=pow  SaturateOnIntegerOverflow=on
  Terminator : Terminator
  Terminator1 : Terminator
  Terminator2 : Terminator
  j(t) : Outport
  wires:
  a [6x1]/1 -> Demux/1
  Constant3/1 -> Math Function4/2
  Add/1 -> j(t)/1
  Demux/4 -> Divide3/2
  t/1 -> Divide4/1, Math Function4/1
  Demux/5 -> Divide4/2
  Demux/6 -> Divide5/2
  Demux/1 -> Terminator/1
  Demux/2 -> Terminator1/1
  Divide3/1 -> Gain2/1
  Divide4/1 -> Gain1/1
  Divide5/1 -> Gain/1
  Gain/1 -> Add/3
  Gain1/1 -> Add/2
  Gain2/1 -> Add/1
  Math Function4/1 -> Divide5/1
  Constant1/1 -> Divide3/1
  Demux/3 -> Terminator2/1

== system ramadan_2022/Supraspinal Level/Subsystem/Swing Leg/Compute Acceleration Profiles with Minimal Jerk Approach/Minimal jerk Hip Roll4/Minimal Jerk Parameters[Movellan] ==
  x0 : Inport
  dx0 : Inport  Port=2
  ddx0 : Inport  Port=3
  xT : Inport  Port=4
  dxT : Inport  Port=5
  ddxT : Inport  Port=6
  T : Inport  Port=7
  Demux : Demux  Outputs=3
  Gain : Gain  Gain=0.5
  Gain1 : Gain  Gain=3
  Gain2 : Gain  Gain=6
  Gain3 : Gain  Gain=4
  Gain4 : Gain  Gain=12
  Gain5 : Gain  Gain=5
  Gain6 : Gain  Gain=20
  Matrix Multiply : Product  Multiplication=Matrix(*)
  Minus : Sum  Inputs=+---
  Minus1 : Sum  Inputs=+--
  Minus2 : Sum  Inputs=+-
  Mux : Mux  Inputs=6
  Mux{1..4} (4 alike) : Mux  Inputs=3
  Pseudoinverse : dspinverses/Pseudoinverse  wanterr=off  SimulateUsing=Code generation
      settings: SourceProductBaseCode=DS
  T{2..5} (4 alike) : Product  Inputs=**
  b : Concatenate  NumInputs=3  Mode=Multidimensional array  ConcatenateDimension=2
  multiply : Product  Inputs=**
  multiply1 : Product  Inputs=**
  multiply2 : Product  Inputs=**
  a : Outport
  wires:
  xT/1 -> Minus/1
  Minus1/1 -> Mux4/2
  T5/1 -> Mux3/1
  multiply1/1 -> Minus1/3
  Gain5/1 -> Mux3/2
  Demux/2 -> Mux/5
  dxT/1 -> Minus1/1
  Demux/3 -> Mux/6
  b/1 -> Pseudoinverse/1
  multiply2/1 -> Minus/3
  Minus2/1 -> Mux4/3
  Gain/1 -> multiply/1, Mux/3
  multiply/1 -> Minus/4
  ddxT/1 -> Minus2/1
  Gain4/1 -> Mux2/3
  Gain6/1 -> Mux3/3
  x0/1 -> Minus/2, Mux/1
  Mux1/1 -> b/1
  Matrix Multiply/1 -> Demux/1
  ddx0/1 -> Minus2/2, multiply1/1, Gain/1
  T2/1 -> Gain1/1, Gain4/1, T3/1, multiply/2
  Gain2/1 -> Mux1/3
  Mux4/1 -> Matrix Multiply/2
  T4/1 -> Mux2/1, Gain5/1, T5/1
  Minus/1 -> Mux4/1
  Pseudoinverse/1 -> Matrix Multiply/1
  Mux2/1 -> b/2
  Gain3/1 -> Mux2/2
  Mux3/1 -> b/3
  Gain1/1 -> Mux1/2
  T/1 -> multiply2/2, multiply1/2, Gain2/1, T5/2, T4/2, T3/2, T2/2, T2/1
  Demux/1 -> Mux/4
  Mux/1 -> a/1
  T3/1 -> Gain6/1, Gain3/1, Mux1/1, T4/1
  dx0/1 -> multiply2/1, Minus1/2, Mux/2

== system ramadan_2022/Supraspinal Level/Subsystem/Swing Leg/Compute Acceleration Profiles with Minimal Jerk Approach/Minimal jerk Knee/Enabled Subsystem ==
  In1 : Inport
  Enable : EnablePort
  Out1 : Outport  VectorParamsAs1DForOutWhenUnconnected=off
  wires:
  In1/1 -> Out1/1

== system ramadan_2022/Supraspinal Level/Subsystem/Swing Leg/Compute Acceleration Profiles with Minimal Jerk Approach/Minimal jerk Knee/Minimal Jerk ==
  t : Inport
  a [6x1] : Inport  Port=2
  Add : Sum  Inputs=3
  Constant1 : Constant
  Constant3 : Constant  Value=2
  Demux : Demux  Outputs=6
  Divide3 : Product  Inputs=**
  Divide4 : Product  Inputs=**
  Divide5 : Product  Inputs=**
  Gain : Gain  Gain=60
  Gain1 : Gain  Gain=24
  Gain2 : Gain  Gain=6
  Math Function4 : Math  Operator=pow  SaturateOnIntegerOverflow=on
  Terminator : Terminator
  Terminator1 : Terminator
  Terminator2 : Terminator
  j(t) : Outport
  wires:
  a [6x1]/1 -> Demux/1
  Constant3/1 -> Math Function4/2
  Add/1 -> j(t)/1
  Demux/4 -> Divide3/2
  t/1 -> Divide4/1, Math Function4/1
  Demux/5 -> Divide4/2
  Demux/6 -> Divide5/2
  Demux/1 -> Terminator/1
  Demux/2 -> Terminator1/1
  Divide3/1 -> Gain2/1
  Divide4/1 -> Gain1/1
  Divide5/1 -> Gain/1
  Gain/1 -> Add/3
  Gain1/1 -> Add/2
  Gain2/1 -> Add/1
  Math Function4/1 -> Divide5/1
  Constant1/1 -> Divide3/1
  Demux/3 -> Terminator2/1

== system ramadan_2022/Supraspinal Level/Subsystem/Swing Leg/Compute Acceleration Profiles with Minimal Jerk Approach/Minimal jerk Knee/Minimal Jerk Parameters [Movellan] ==
  x0 : Inport
  dx0 : Inport  Port=2
  ddx0 : Inport  Port=3
  xT : Inport  Port=4
  dxT : Inport  Port=5
  ddxT : Inport  Port=6
  T : Inport  Port=7
  Demux : Demux  Outputs=3
  Gain : Gain  Gain=0.5
  Gain1 : Gain  Gain=3
  Gain2 : Gain  Gain=6
  Gain3 : Gain  Gain=4
  Gain4 : Gain  Gain=12
  Gain5 : Gain  Gain=5
  Gain6 : Gain  Gain=20
  Matrix Multiply : Product  Multiplication=Matrix(*)
  Minus : Sum  Inputs=+---
  Minus1 : Sum  Inputs=+--
  Minus2 : Sum  Inputs=+-
  Mux : Mux  Inputs=6
  Mux{1..4} (4 alike) : Mux  Inputs=3
  Pseudoinverse : dspinverses/Pseudoinverse  wanterr=off  SimulateUsing=Code generation
      settings: SourceProductBaseCode=DS
  T{2..5} (4 alike) : Product  Inputs=**
  b : Concatenate  NumInputs=3  Mode=Multidimensional array  ConcatenateDimension=2
  multiply : Product  Inputs=**
  multiply1 : Product  Inputs=**
  multiply2 : Product  Inputs=**
  a : Outport
  wires:
  xT/1 -> Minus/1
  Minus1/1 -> Mux4/2
  T5/1 -> Mux3/1
  multiply1/1 -> Minus1/3
  Gain5/1 -> Mux3/2
  Demux/2 -> Mux/5
  dxT/1 -> Minus1/1
  Demux/3 -> Mux/6
  b/1 -> Pseudoinverse/1
  multiply2/1 -> Minus/3
  Minus2/1 -> Mux4/3
  Gain/1 -> multiply/1, Mux/3
  multiply/1 -> Minus/4
  ddxT/1 -> Minus2/1
  Gain4/1 -> Mux2/3
  Gain6/1 -> Mux3/3
  x0/1 -> Minus/2, Mux/1
  Mux1/1 -> b/1
  Matrix Multiply/1 -> Demux/1
  ddx0/1 -> Minus2/2, multiply1/1, Gain/1
  T2/1 -> Gain1/1, Gain4/1, T3/1, multiply/2
  Gain2/1 -> Mux1/3
  Mux4/1 -> Matrix Multiply/2
  T4/1 -> Mux2/1, Gain5/1, T5/1
  Minus/1 -> Mux4/1
  Pseudoinverse/1 -> Matrix Multiply/1
  Mux2/1 -> b/2
  Gain3/1 -> Mux2/2
  Mux3/1 -> b/3
  Gain1/1 -> Mux1/2
  T/1 -> multiply2/2, multiply1/2, Gain2/1, T5/2, T4/2, T3/2, T2/2, T2/1
  Demux/1 -> Mux/4
  Mux/1 -> a/1
  T3/1 -> Gain6/1, Gain3/1, Mux1/1, T4/1
  dx0/1 -> multiply2/1, Minus1/2, Mux/2

== system ramadan_2022/Supraspinal Level/Subsystem/Swing Leg/Compute Acceleration Profiles with Minimal Jerk Approach1/ Timer Phase 1/Resettable Subsystem ==
  In1 : Inport
  Enable : EnablePort  ZeroCross=off
  Out1 : Outport
  wires:
  In1/1 -> Out1/1

== system ramadan_2022/Supraspinal Level/Subsystem/Swing Leg/Compute Acceleration Profiles with Minimal Jerk Approach1/ Timer Phase 2/Resettable Subsystem ==
  In1 : Inport
  Enable : EnablePort  ZeroCross=off
  Out1 : Outport
  wires:
  In1/1 -> Out1/1

== system ramadan_2022/Supraspinal Level/Subsystem/Swing Leg/Compute Acceleration Profiles with Minimal Jerk Approach1/ Timer Phase 3/Resettable Subsystem ==
  In1 : Inport
  Enable : EnablePort  ZeroCross=off
  Out1 : Outport
  wires:
  In1/1 -> Out1/1

== system ramadan_2022/Supraspinal Level/Subsystem/Swing Leg/Compute Acceleration Profiles with Minimal Jerk Approach1/ Timer Phase 4/Resettable Subsystem ==
  In1 : Inport
  Enable : EnablePort  ZeroCross=off
  Out1 : Outport
  wires:
  In1/1 -> Out1/1

== system ramadan_2022/Supraspinal Level/Subsystem/Swing Leg/Compute Acceleration Profiles with Minimal Jerk Approach1/Minimal jerk Hip Roll4/Minimal Jerk ==
  t : Inport
  a [6x1] : Inport  Port=2
  Add : Sum  Inputs=3
  Constant1 : Constant
  Constant3 : Constant  Value=2
  Demux : Demux  Outputs=6
  Divide3 : Product  Inputs=**
  Divide4 : Product  Inputs=**
  Divide5 : Product  Inputs=**
  Gain : Gain  Gain=60
  Gain1 : Gain  Gain=24
  Gain2 : Gain  Gain=6
  Math Function4 : Math  Operator=pow  SaturateOnIntegerOverflow=on
  Terminator : Terminator
  Terminator1 : Terminator
  Terminator2 : Terminator
  j(t) : Outport
  wires:
  a [6x1]/1 -> Demux/1
  Constant3/1 -> Math Function4/2
  Add/1 -> j(t)/1
  Demux/4 -> Divide3/2
  t/1 -> Divide4/1, Math Function4/1
  Demux/5 -> Divide4/2
  Demux/6 -> Divide5/2
  Demux/1 -> Terminator/1
  Demux/2 -> Terminator1/1
  Divide3/1 -> Gain2/1
  Divide4/1 -> Gain1/1
  Divide5/1 -> Gain/1
  Gain/1 -> Add/3
  Gain1/1 -> Add/2
  Gain2/1 -> Add/1
  Math Function4/1 -> Divide5/1
  Constant1/1 -> Divide3/1
  Demux/3 -> Terminator2/1

== system ramadan_2022/Supraspinal Level/Subsystem/Swing Leg/Compute Acceleration Profiles with Minimal Jerk Approach1/Minimal jerk Hip Roll4/Minimal Jerk Parameters[Movellan] ==
  x0 : Inport
  dx0 : Inport  Port=2
  ddx0 : Inport  Port=3
  xT : Inport  Port=4
  dxT : Inport  Port=5
  ddxT : Inport  Port=6
  T : Inport  Port=7
  Demux : Demux  Outputs=3
  Gain : Gain  Gain=0.5
  Gain1 : Gain  Gain=3
  Gain2 : Gain  Gain=6
  Gain3 : Gain  Gain=4
  Gain4 : Gain  Gain=12
  Gain5 : Gain  Gain=5
  Gain6 : Gain  Gain=20
  Matrix Multiply : Product  Multiplication=Matrix(*)
  Minus : Sum  Inputs=+---
  Minus1 : Sum  Inputs=+--
  Minus2 : Sum  Inputs=+-
  Mux : Mux  Inputs=6
  Mux{1..4} (4 alike) : Mux  Inputs=3
  Pseudoinverse : dspinverses/Pseudoinverse  wanterr=off  SimulateUsing=Code generation
      settings: SourceProductBaseCode=DS
  T{2..5} (4 alike) : Product  Inputs=**
  b : Concatenate  NumInputs=3  Mode=Multidimensional array  ConcatenateDimension=2
  multiply : Product  Inputs=**
  multiply1 : Product  Inputs=**
  multiply2 : Product  Inputs=**
  a : Outport
  wires:
  xT/1 -> Minus/1
  Minus1/1 -> Mux4/2
  T5/1 -> Mux3/1
  multiply1/1 -> Minus1/3
  Gain5/1 -> Mux3/2
  Demux/2 -> Mux/5
  dxT/1 -> Minus1/1
  Demux/3 -> Mux/6
  b/1 -> Pseudoinverse/1
  multiply2/1 -> Minus/3
  Minus2/1 -> Mux4/3
  Gain/1 -> multiply/1, Mux/3
  multiply/1 -> Minus/4
  ddxT/1 -> Minus2/1
  Gain4/1 -> Mux2/3
  Gain6/1 -> Mux3/3
  x0/1 -> Minus/2, Mux/1
  Mux1/1 -> b/1
  Matrix Multiply/1 -> Demux/1
  ddx0/1 -> Minus2/2, multiply1/1, Gain/1
  T2/1 -> Gain1/1, Gain4/1, T3/1, multiply/2
  Gain2/1 -> Mux1/3
  Mux4/1 -> Matrix Multiply/2
  T4/1 -> Mux2/1, Gain5/1, T5/1
  Minus/1 -> Mux4/1
  Pseudoinverse/1 -> Matrix Multiply/1
  Mux2/1 -> b/2
  Gain3/1 -> Mux2/2
  Mux3/1 -> b/3
  Gain1/1 -> Mux1/2
  T/1 -> multiply2/2, multiply1/2, Gain2/1, T5/2, T4/2, T3/2, T2/2, T2/1
  Demux/1 -> Mux/4
  Mux/1 -> a/1
  T3/1 -> Gain6/1, Gain3/1, Mux1/1, T4/1
  dx0/1 -> multiply2/1, Minus1/2, Mux/2

== system ramadan_2022/Supraspinal Level/Subsystem/Swing Leg/Compute Acceleration Profiles with Minimal Jerk Approach1/Minimal jerk Leg Angle/Enabled Subsystem ==
  In1 : Inport
  Enable : EnablePort
  Out1 : Outport  VectorParamsAs1DForOutWhenUnconnected=off
  wires:
  In1/1 -> Out1/1
